simulink model "Main_Model_v0"  (R2025a)
settings: Solver=VariableStepAuto  StartTime=0.0  StopTime=800  RelTol=1e-3  AbsTol=1e-3
values from neighbouring files (symbols this model uses):
  area_air = 0.0353    [air_params.m]
  cp_air = 1005    [air_params.m]
  eta_map = [nan nan nan nan nan nan nan nan nan nan nan nan ... (240 elements, 15x16)]    [motor efficiency map.mat]
  HC_min = 1    [air_params.m]
  HC_nom = 266.43    [air_params.m]
  rho_air = 1.225    [air_params.m]
  speed_bp_rpm = [500 1000 1500 2000 2500 3000 3500 4000 4500 5000 5500 6000 ... (16 elements, 1x16)]    [motor efficiency map.mat]
  torque_bp_Nm = [0 25 50 75 100 125 150 175 200 225 250 275 ... (15 elements, 1x15)]    [motor efficiency map.mat]
  vel_air_nom = 0.18878    [air_params.m]
libraries: fl_lib x26, nesl_utility x14, SimscapeFluids_lib x3
(part 2 of 3)

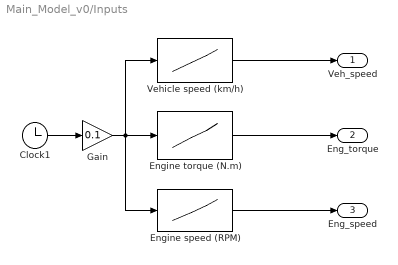
== system Main_Model_v0/Inputs ==
  Clock1 : Clock
  Engine speed (RPM) : Lookup  InputValues=|  Table=|  LookUpMeth=Interpolation-Use End Values
      | [0
      | 1
      | 2
      | 3
      | 4
      | 5
      | 6
      | 7
      | 8
      | 9
      | 10
      | 11
      | 12
      | 13
      | 14
      | 15
      | 16
      | 17
      | 18
      | 19
      | 20
      | 21
      | 22
      | 23
      | 24
      | 25
      | 26
      | 27
      | 28
      | 29
      | 30
      | 31
      | 32
      | 33
      | 34
      | 35
      | 36
      | 37
      | 38
      | 39
      | 40
      | 41
      | 42
      | 43
      | 44
      | 45
      | 46
      | 47
      | 48
      | 49
      | 50
      | 51
      | 52
      | 53
      | 54
      | 55
      | 56
      | 57
      | 58
      | 59
      | 61
      | 62
      | 63
      | 64
      | 65
      | 66
      | 67
      | 68
      | 69
      | 70
      | 71
      | 72
      | 73
      | 74
      | 75
      | 76
      | 77
      | 78
      | 79
      | 80
      | 81
      | 82
      | 83
      | 84
      | 85
      | 86
      | 87
      | 88
      | 89
      | 90
      | 91
      | 92
      | 93
      | 94
      | 95
      | 96
      | 97
      | 98
      | 99
      | 100
      | 101
      | 102
      | 103
      | 104
      | 105
      | 106
      | 107
      | 108
      | 109
      | 110
      | 111
      | 112
      | 113
      | 114
      | 115
      | 116
      | 117
      | 118
      | 119
      | 120
      | 121
      | 122
      | 123
      | 124
      | 125
      | 126
      | 127
      | 129
      | 130
      | 131
      | 132
      | 133
      | 134
      | 135
      | 136
      | 137
      | 138
      | 139
      | 140
      | 141
      | 142
      | 143
      | 144
      | 145
      | 146
      | 147
      | 148
      | 149
      | 150
      | 151
      | 152
      | 153
      | 154
      | 155
      | 156
      | 157
      | 158
      | 159
      | 160
      | 161
      | 162
      | 163
      | 164
      | 165
      | 166
      | 167
      | 168
      | 169
      | 170
      | 171
      | 172
      | 173
      | 174
      | 175
      | 176
      | 177
      | 178
      | 179
      | 180
      | 182
      | 183
      | 184
      | 185
      | 186
      | 187
      | 188
      | 189
      | 190
      | 191
      | 192
      | 193
      | 194
      | 195
      | 196
      | 197
      | 198
      | 199
      | 200
      | 201
      | 202
      | 203
      | 204
      | 205
      | 206
      | 207
      | 208
      | 209
      | 210
      | 211
      | 212
      | 213
      | 214
      | 215
      | 216
      | 217
      | 218
      | 219
      | 220
      | 221
      | 222
      | 223
      | 224
      | 225
      | 226
      | 227
      | 228
      | 229
      | 230
      | 231
      | 232
      | 233
      | 234
      | 235
      | 236
      | 237
      | 238
      | 239
      | 240
      | 241
      | 242
      | 243
      | 244
      | 245
      | 246
      | 247
      | 248
      | 249
      | 250
      | 251
      | 252
      | 253
      | 254
      | 255
      | 256
      | 257
      | 258
      | 259
      | 260
      | 261
      | 262
      | 263
      | 264
      | 265
      | 266
      | 267
      | 268
      | 269
      | 270
      | 271
      | 272
      | 273
      | 274
      | 275
      | 276
      | 277
      | 278
      | 279
      | 280
      | 281
      | 282
      | 283
      | 284
      | 285
      | 286
      | 287
      | 288
      | 289
      | 290
      | 291
      | 292
      | 293
      | 294
      | 295
      | 296
      | 297
      | 298
      | 299
      | 300
      | 301
      | 302
      | 303
      | 304
      | 305
      | 306
      | 307
      | 308
      | 309
      | 310
      | 311
      | 312
      | 313
      | 314
      | 315
      | 316
      | 317
      | 318
      | 319
      | 320
      | 321
      | 322
      | 323
      | 324
      | 325
      | 326
      | 327
      | 328
      | 329
      | 330
      | 331
      | 332
      | 333
      | 335
      | 336
      | 337
      | 338
      | 339
      | 340
      | 341
      | 342
      | 343
      | 344
      | 345
      | 346
      | 347
      | 348
      | 349
      | 350
      | 351
      | 352
      | 353
      | 354
      | 355
      | 356
      | 357
      | 358
      | 359
      | 360
      | 361
      | 362
      | 363
      | 364
      | 365
      | 366
      | 367
      | 368
      | 369
      | 370
      | 371
      | 372
      | 373
      | 374
      | 375
      | 377
      | 378
      | 379
      | 380
      | 381
      | 382
      | 383
      | 384
      | 385
      | 386
      | 387
      | 388
      | 389
      | 390
      | 391
      | 392
      | 393
      | 394
      | 395
      | 396
      | 397
      | 398
      | 399
      | 400
      | 401
      | 402
      | 403
      | 404
      | 405
      | 406
      | 407
      | 408
      | 409
      | 410
      | 411
      | 412
      | 413
      | 414
      | 415
      | 416
      | 417
      | 418
      | 419
      | 420
      | 421
      | 422
      | 423
      | 424
      | 425
      | 426
      | 427
      | 428
      | 429
      | 430
      | 431
      | 432
      | 433
      | 434
      | 435
      | 436
      | 437
      | 438
      | 439
      | 440
      | 441
      | 442
      | 443
      | 444
      | 445
      | 446
      | 447
      | 448
      | 449
      | 450
      | 451
      | 452
      | 453
      | 454
      | 455
      | 456
      | 457
      | 458
      | 459
      | 460
      | 461
      | 462
      | 463
      | 464
      | 465
      | 466
      | 467
      | 468
      | 469
      | 470
      | 471
      | 472
      | 473
      | 474
      | 475
      | 476
      | 477
      | 478
      | 479
      | 480
      | 481
      | 482
      | 483
      | 484
      | 485
      | 486
      | 487
      | 488
      | 489
      | 490
      | 491
      | 492
      | 493
      | 494
      | 495
      | 496
      | 497
      | 498
      | 499
      | 500
      | 501
      | 502
      | 503
      | 504
      | 505
      | 506
      | 507
      | 508
      | 509
      | 510
      | 511
      | 512
      | 513
      | 514
      | 515
      | 516
      | 517
      | 518
      | 519
      | 520
      | 521
      | 522
      | 523
      | 524
      | 525
      | 526
      | 527
      | 528
      | 530
      | 531
      | 532
      | 533
      | 534
      | 535
      | 536
      | 537
      | 538
      | 539
      | 540
      | 541
      | 542
      | 543
      | 544
      | 545
      | 546
      | 547
      | 548
      | 549
      | 550
      | 551
      | 552
      | 553
      | 554
      | 555
      | 556
      | 557
      | 558
      | 559
      | 560
      | 561
      | 562
      | 563
      | 564
      | 565
      | 566
      | 567
      | 568
      | 569
      | 570
      | 572
      | 573
      | 574
      | 575
      | 576
      | 577
      | 578
      | 579
      | 580
      | 581
      | 582
      | 583
      | 584
      | 585
      | 586
      | 587
      | 588
      | 589
      | 590
      | 591
      | 592
      | 593
      | 594
      | 595
      | 596
      | 597
      | 598
      | 599
      | 600
      | 601
      | 602
      | 603
      | 604
      | 605
      | 606
      | 607
      | 608
      | 609
      | 610
      | 611
      | 612
      | 613
      | 614
      | 615
      | 616
      | 617
      | 618
      | 619
      | 620
      | 621
      | 622
      | 623
      | 624
      | 625
      | 626
      | 627
      | 628
      | 629
      | 630
      | 631
      | 632
      | 633
      | 634
      | 635
      | 636
      | 637
      | 638
      | 639
      | 640
      | 641
      | 642
      | 643
      | 644
      | 645
      | 646
      | 647
      | 648
      | 649
      | 650
      | 651
      | 652
      | 653
      | 654
      | 655
      | 656
      | 657
      | 658
      | 659
      | 660
      | 661
      | 662
      | 663
      | 664
      | 665
      | 666
      | 667
      | 668
      | 669
      | 670
      | 671
      | 672
      | 673
      | 674
      | 675
      | 676
      | 677
      | 678
      | 679
      | 680
      | 681
      | 682
      | 683
      | 684
      | 685
      | 686
      | 687
      | 688
      | 689
      | 690
      | 691
      | 692
      | 693
      | 694
      | 695
      | 696
      | 697
      | 698
      | 699
      | 700
      | 701
      | 702
      | 703
      | 704
      | 705
      | 706
      | 707
      | 708
      | 709
      | 710
      | 711
      | 712
      | 713
      | 714
      | 715
      | 716
      | 717
      | 718
      | 719
      | 720
      | 721
      | 722
      | 723
      | 725
      | 726
      | 727
      | 728
      | 729
      | 730
      | 731
      | 732
      | 733
      | 734
      | 735
      | 736
      | 737
      | 738
      | 739
      | 740
      | 741
      | 742
      | 743
      | 744
      | 745
      | 746
      | 747
      | 748
      | 749
      | 750
      | 751
      | 752
      | 753
      | 754
      | 755
      | 756
      | 757
      | 758
      | 759
      | 760
      | 761
      | 762
      | 763
      | 764
      | 765
      | 766
      | 767
      | 768
      | 769
      | 770
      | 771
      | 772
      | 773
      | 774
      | 775
      | 776
      | 777
      | 778
      | 779
      | 780
      | 781
      | 782
      | 783
      | 784
      | 785
      | 786
      | 787
      | 788
      | 789
      | 790
      | 791
      | 792
      | 793
      | 794
      | 795
      | 796
      | 797
      | 798
      | 799
      | 800
      | 801
      | 802
      | 803
      | 804
      | 805
      | 806
      | 807
      | 808
      | 809
      | 810
      | 811
      | 812
      | 813
      | 814
      | 815
      | 816
      | 817
      | 818
      | 819
      | 820
      | 821
      | 823
      | 824
      | 825
      | 826
      | 827
      | 828
      | 829
      | 830
      | 831
      | 833
      | 834
      | 835
      | 836
      | 837
      | 838
      | 839
      | 840
      | 841
      | 842
      | 843
      | 844
      | 845
      | 846
      | 848
      | 849
      | 850
      | 851
      | 852
      | 853
      | 854
      | 855
      | 856
      | 857
      | 858
      | 859
      | 860
      | 861
      | 862
      | 863
      | 864
      | 865
      | 866
      | 867
      | 868
      | 869
      | 870
      | 871
      | 872
      | 873
      | 874
      | 875
      | 876
      | 877
      | 878
      | 879
      | 880
      | 881
      | 882
      | 883
      | 884
      | 885
      | 886
      | 887
      | 888
      | 889
      | 890
      | 891
      | 892
      | 893
      | 894
      | 895
      | 896
      | 897
      | 898
      | 899
      | 901
      | 902
      | 903
      | 904
      | 905
      | 906
      | 907
      | 908
      | 909
      | 910
      | 911
      | 912
      | 913
      | 914
      | 915
      | 916
      | 917
      | 918
      | 919
      | 920
      | 921
      | 922
      | 923
      | 924
      | 925
      | 926
      | 927
      | 928
      | 929
      | 930
      | 931
      | 932
      | 933
      | 934
      | 935
      | 936
      | 937
      | 938
      | 939
      | 940
      | 941
      | 942
      | 943
      | 944
      | 945
      | 946
      | 947
      | 948
      | 949
      | 950
      | 951
      | 952
      | 953
      | 954
      | 955
      | 956
      | 957
      | 958
      | 959
      | 960
      | 961
      | 962
      | 963
      | 964
      | 965
      | 966
      | 967
      | 968
      | 969
      | 970
      | 971
      | 972
      | 973
      | 974
      | 975
      | 976
      | 977
      | 978
      | 979
      | 980
      | 981
      | 982
      | 983
      | 984
      | 985
      | 986
      | 988
      | 989
      | 990
      | 991
      | 992
      | 993
      | 994
      | 995
      | 996
      | 997
      | 998
      | 999
      | 1000
      | 1001
      | 1002
      | 1003
      | 1004
      | 1005
      | 1006
      | 1007
      | 1008
      | 1009
      | 1010
      | 1011
      | 1012
      | 1013
      | 1014
      | 1015
      | 1016
      | 1017
      | 1018
      | 1019
      | 1020
      | 1021
      | 1022
      | 1023
      | 1024
      | 1025
      | 1026
      | 1027
      | 1028
      | 1029
      | 1030
      | 1031
      | 1032
      | 1033
      | 1034
      | 1035
      | 1036
      | 1037
      | 1038
      | 1039
      | 1040
      | 1041
      | 1042
      | 1043
      | 1044
      | 1045
      | 1046
      | 1047
      | 1048
      | 1049
      | 1050
      | 1051
      | 1052
      | 1053
      | 1054
      | 1055
      | 1056
      | 1057
      | 1058
      | 1059
      | 1060
      | 1061
      | 1062
      | 1063
      | 1064
      | 1065
      | 1066
      | 1067
      | 1068
      | 1069
      | 1070
      | 1071
      | 1072
      | 1073
      | 1074
      | 1075
      | 1076
      | 1077
      | 1078
      | 1079
      | 1080
      | 1081
      | 1082
      | 1083
      | 1084
      | 1085
      | 1086
      | 1087
      | 1088
      | 1089
      | 1090
      | 1091
      | 1092
      | 1093
      | 1094
      | 1095
      | 1096
      | 1097
      | 1098
      | 1099
      | 1100
      | 1101
      | 1102
      | 1103
      | 1104
      | 1105
      | 1106
      | 1107
      | 1108
      | 1109
      | 1110
      | 1111
      | 1112
      | 1113
      | 1114
      | 1115
      | 1116
      | 1117
      | 1118
      | 1119
      | 1120
      | 1121
      | 1122
      | 1123
      | 1124
      | 1125
      | 1126
      | 1127
      | 1128
      | 1129
      | 1130
      | 1131
      | 1132
      | 1133
      | 1134
      | 1135
      | 1136
      | 1137
      | 1138
      | 1139
      | 1140
      | 1141
      | 1142
      | 1143
      | 1144
      | 1145
      | 1146
      | 1147
      | 1148
      | 1149
      | 1150
      | 1151
      | 1152
      | 1153
      | 1154
      | 1155
      | 1156
      | 1157
      | 1158
      | 1159
      | 1160
      | 1161
      | 1162
      | 1163
      | 1164
      | 1165
      | 1166
      | 1167
      | 1168
      | 1169
      | 1170
      | 1171
      | 1172
      | 1173
      | 1174
      | 1175
      | 1176
      | 1177
      | 1178
      | 1179
      | 1180
      | 1181
      | 1182
      | 1183
      | 1184
      | 1185
      | 1186
      | 1187
      | 1188
      | 1189
      | 1190
      | 1191
      | 1192
      | 1193
      | 1194
      | 1195
      | 1196
      | 1197
      | 1198
      | 1199
      | 1200
      | 1201
      | 1202
      | 1203
      | 1204
      | 1205]
      | [10
      | 10
      | 10
      | 10
      | 806
      | 1376
      | 1306
      | 1251
      | 1223
      | 1214
      | 1207
      | 1214
      | 1234
      | 1188
      | 1189
      | 1029
      | 1032
      | 978
      | 970
      | 1350
      | 1799
      | 1957
      | 1948
      | 1935
      | 1915
      | 1894
      | 1875
      | 1851
      | 1757
      | 1500
      | 1158
      | 1074
      | 1025
      | 991
      | 973
      | 978
      | 974
      | 970
      | 980
      | 979
      | 972
      | 954
      | 984
      | 975
      | 972
      | 971
      | 976
      | 958
      | 956
      | 963
      | 974
      | 973
      | 963
      | 1017
      | 1026
      | 1043
      | 1036
      | 1300
      | 1752
      | 1910
      | 988
      | 1170
      | 1523
      | 1747
      | 1911
      | 2117
      | 2171
      | 2172
      | 2167
      | 2171
      | 2174
      | 2167
      | 2168
      | 2163
      | 2161
      | 2158
      | 2148
      | 2150
      | 2139
      | 2140
      | 2135
      | 2130
      | 2125
      | 2122
      | 2117
      | 2109
      | 2111
      | 2106
      | 2099
      | 2019
      | 1896
      | 1722
      | 1547
      | 1372
      | 1204
      | 1035
      | 986
      | 963
      | 941
      | 941
      | 935
      | 925
      | 930
      | 919
      | 915
      | 923
      | 922
      | 931
      | 911
      | 926
      | 933
      | 913
      | 917
      | 930
      | 920
      | 915
      | 924
      | 914
      | 916
      | 916
      | 921
      | 932
      | 1028
      | 1015
      | 1282
      | 1742
      | 1900
      | 997
      | 1123
      | 1375
      | 1488
      | 1711
      | 1864
      | 1976
      | 2128
      | 2289
      | 2296
      | 1551
      | 1593
      | 1684
      | 1799
      | 1902
      | 1978
      | 2071
      | 2138
      | 2198
      | 2248
      | 2264
      | 2268
      | 2272
      | 2268
      | 2264
      | 2262
      | 2259
      | 2258
      | 2252
      | 2249
      | 2250
      | 2199
      | 2142
      | 2069
      | 1979
      | 1905
      | 1828
      | 1747
      | 1687
      | 1610
      | 1622
      | 1610
      | 1602
      | 1602
      | 1598
      | 1597
      | 1594
      | 1603
      | 1597
      | 1590
      | 1598
      | 1603
      | 2234
      | 2150
      | 1948
      | 1743
      | 1518
      | 1307
      | 1098
      | 967
      | 933
      | 907
      | 879
      | 873
      | 880
      | 876
      | 875
      | 878
      | 868
      | 871
      | 869
      | 859
      | 854
      | 867
      | 874
      | 873
      | 852
      | 864
      | 867
      | 872
      | 810
      | 795
      | 1005
      | 989
      | 1327
      | 1805
      | 1973
      | 1956
      | 1939
      | 1922
      | 1893
      | 1874
      | 1845
      | 1755
      | 1497
      | 900
      | 877
      | 863
      | 858
      | 869
      | 850
      | 862
      | 856
      | 850
      | 846
      | 858
      | 849
      | 844
      | 858
      | 850
      | 852
      | 863
      | 847
      | 849
      | 855
      | 840
      | 859
      | 855
      | 799
      | 783
      | 1018
      | 1053
      | 1297
      | 1733
      | 1917
      | 1013
      | 952
      | 1184
      | 1515
      | 1756
      | 1911
      | 2105
      | 2170
      | 2172
      | 2174
      | 2172
      | 2175
      | 2166
      | 2167
      | 2165
      | 2161
      | 2156
      | 2148
      | 2148
      | 2138
      | 2142
      | 2137
      | 2130
      | 2124
      | 2121
      | 2113
      | 2107
      | 2112
      | 2105
      | 2099
      | 2030
      | 1895
      | 1717
      | 1551
      | 1367
      | 1200
      | 1024
      | 922
      | 897
      | 867
      | 835
      | 834
      | 815
      | 837
      | 821
      | 820
      | 812
      | 819
      | 823
      | 811
      | 831
      | 819
      | 812
      | 833
      | 825
      | 810
      | 828
      | 824
      | 807
      | 831
      | 821
      | 793
      | 803
      | 1020
      | 1043
      | 1282
      | 1751
      | 1912
      | 994
      | 1000
      | 1132
      | 1358
      | 1524
      | 1704
      | 1850
      | 1994
      | 2125
      | 2282
      | 2295
      | 1590
      | 1688
      | 1780
      | 1885
      | 1983
      | 2065
      | 2136
      | 2204
      | 2255
      | 2260
      | 2266
      | 2266
      | 2269
      | 2269
      | 2266
      | 2258
      | 2262
      | 2259
      | 2250
      | 2246
      | 2212
      | 2123
      | 2057
      | 1983
      | 1906
      | 1840
      | 1765
      | 1684
      | 1616
      | 1622
      | 1603
      | 1599
      | 1606
      | 1599
      | 1592
      | 1603
      | 1597
      | 1595
      | 1592
      | 1604
      | 1595
      | 2223
      | 2144
      | 1955
      | 1726
      | 1522
      | 1313
      | 1105
      | 929
      | 877
      | 831
      | 826
      | 799
      | 797
      | 786
      | 803
      | 788
      | 790
      | 792
      | 788
      | 783
      | 792
      | 793
      | 780
      | 781
      | 793
      | 796
      | 777
      | 801
      | 787
      | 816
      | 970
      | 1021
      | 1317
      | 1807
      | 1976
      | 1951
      | 1934
      | 1919
      | 1889
      | 1871
      | 1851
      | 1758
      | 1497
      | 869
      | 806
      | 784
      | 791
      | 796
      | 786
      | 781
      | 789
      | 793
      | 790
      | 779
      | 794
      | 789
      | 788
      | 785
      | 779
      | 791
      | 784
      | 789
      | 777
      | 782
      | 793
      | 791
      | 790
      | 813
      | 1005
      | 1044
      | 1295
      | 1730
      | 1912
      | 1003
      | 960
      | 1187
      | 1499
      | 1785
      | 1908
      | 2123
      | 2169
      | 2168
      | 2174
      | 2173
      | 2173
      | 2166
      | 2162
      | 2163
      | 2162
      | 2154
      | 2145
      | 2147
      | 2139
      | 2139
      | 2138
      | 2133
      | 2128
      | 2115
      | 2116
      | 2115
      | 2111
      | 2104
      | 2101
      | 2027
      | 1893
      | 1715
      | 1548
      | 1369
      | 1197
      | 1026
      | 884
      | 839
      | 809
      | 800
      | 780
      | 779
      | 782
      | 779
      | 781
      | 780
      | 780
      | 781
      | 781
      | 786
      | 780
      | 773
      | 766
      | 771
      | 775
      | 779
      | 761
      | 778
      | 782
      | 772
      | 794
      | 817
      | 983
      | 1054
      | 1289
      | 1759
      | 1907
      | 992
      | 997
      | 1150
      | 1369
      | 1486
      | 1708
      | 1847
      | 1968
      | 2133
      | 2283
      | 2266
      | 1586
      | 1694
      | 1810
      | 1917
      | 1994
      | 2076
      | 2143
      | 2209
      | 2265
      | 2266
      | 2257
      | 2268
      | 2273
      | 2266
      | 2267
      | 2256
      | 2260
      | 2255
      | 2252
      | 2243
      | 2222
      | 2118
      | 2057
      | 1972
      | 1900
      | 1841
      | 1758
      | 1686
      | 1609
      | 1616
      | 1611
      | 1600
      | 1602
      | 1604
      | 1595
      | 1596
      | 1601
      | 1597
      | 1597
      | 1593
      | 1599
      | 2236
      | 2151
      | 1947
      | 1738
      | 1514
      | 1312
      | 1100
      | 931
      | 848
      | 813
      | 801
      | 791
      | 770
      | 765
      | 774
      | 752
      | 778
      | 757
      | 763
      | 774
      | 750
      | 771
      | 766
      | 754
      | 772
      | 754
      | 762
      | 766
      | 803
      | 812
      | 988
      | 981
      | 1332
      | 1823
      | 1976
      | 1952
      | 1936
      | 1916
      | 1897
      | 1877
      | 1849
      | 1768
      | 1492
      | 839
      | 777
      | 763
      | 753
      | 754
      | 763
      | 764
      | 750
      | 746
      | 743
      | 761
      | 759
      | 758
      | 751
      | 748
      | 767
      | 753
      | 753
      | 768
      | 764
      | 756
      | 770
      | 756
      | 809
      | 811
      | 975
      | 1049
      | 1297
      | 1733
      | 1913
      | 996
      | 958
      | 1178
      | 1511
      | 1786
      | 1917
      | 2120
      | 2170
      | 2173
      | 2174
      | 2170
      | 2172
      | 2164
      | 2165
      | 2167
      | 2164
      | 2157
      | 2146
      | 2152
      | 2135
      | 2140
      | 2136
      | 2131
      | 2131
      | 2121
      | 2113
      | 2112
      | 2110
      | 2105
      | 2097
      | 2035
      | 1882
      | 1713
      | 1551
      | 1374
      | 1207
      | 1034
      | 875
      | 822
      | 790
      | 773
      | 758
      | 742
      | 754
      | 749
      | 750
      | 758
      | 764
      | 746
      | 759
      | 747
      | 756
      | 751
      | 740
      | 741
      | 742
      | 740
      | 733
      | 733
      | 747
      | 757
      | 805
      | 814
      | 975
      | 1050
      | 1239
      | 1725
      | 1905
      | 984
      | 983
      | 1176
      | 1303
      | 1537
      | 1671
      | 1830
      | 1991
      | 2145
      | 2266
      | 2295
      | 1593
      | 1719
      | 1835
      | 1930
      | 2004
      | 2048
      | 2121
      | 2188
      | 2263
      | 2268
      | 2266
      | 2272
      | 2262
      | 2267
      | 2260
      | 2266
      | 2255
      | 2249
      | 2240
      | 2242
      | 2220
      | 2140
      | 2072
      | 1975
      | 1907
      | 1829
      | 1748
      | 1682
      | 1606
      | 1618
      | 1601
      | 1604
      | 1596
      | 1598
      | 1599
      | 1595
      | 1594
      | 1599
      | 1597
      | 1597
      | 1595
      | 1558
      | 2243
      | 2159
      | 1939
      | 1742
      | 1523
      | 1305
      | 1096
      | 925
      | 838
      | 791
      | 781
      | 772
      | 762
      | 755
      | 743
      | 746
      | 750
      | 744
      | 736
      | 747
      | 738
      | 745
      | 751
      | 744
      | 745
      | 756
      | 754
      | 755
      | 760
      | 754
      | 757
      | 753
      | 749
      | 742
      | 751
      | 748
      | 756
      | 829
      | 828
      | 1016
      | 1040
      | 1098
      | 1456
      | 1804
      | 1023
      | 1011
      | 1198
      | 1343
      | 1470
      | 1600
      | 1732
      | 1837
      | 2003
      | 2122
      | 2292
      | 1608
      | 1702
      | 1793
      | 1837
      | 1920
      | 1999
      | 2057
      | 2158
      | 2252
      | 1691
      | 1748
      | 1827
      | 1846
      | 1906
      | 1925
      | 2000
      | 2028
      | 2086
      | 2121
      | 2189
      | 2208
      | 2265
      | 2302
      | 1808
      | 1828
      | 1828
      | 1830
      | 1828
      | 1836
      | 1837
      | 1821
      | 1823
      | 1816
      | 1825
      | 1824
      | 1835
      | 1833
      | 1838
      | 1834
      | 1825
      | 1821
      | 1816
      | 1826
      | 1823
      | 1833
      | 1829
      | 1835
      | 1834
      | 1838
      | 1833
      | 1815
      | 1814
      | 1817
      | 1823
      | 1820
      | 1834
      | 1830
      | 1835
      | 1833
      | 1836
      | 1833
      | 1836
      | 1830
      | 1826
      | 1823
      | 1817
      | 1822
      | 1817
      | 1819
      | 1817
      | 1830
      | 1795
      | 1744
      | 1698
      | 1625
      | 1929
      | 1852
      | 1778
      | 1702
      | 1712
      | 1692
      | 1691
      | 1685
      | 1684
      | 1683
      | 1688
      | 1686
      | 1683
      | 1680
      | 1681
      | 1681
      | 1678
      | 1684
      | 1689
      | 1688
      | 1688
      | 1684
      | 1685
      | 1679
      | 1677
      | 1685
      | 1689
      | 1684
      | 1682
      | 1683
      | 1680
      | 1685
      | 1692
      | 1685
      | 1685
      | 1682
      | 1684
      | 1690
      | 1683
      | 1684
      | 1680
      | 1689
      | 1691
      | 1687
      | 1682
      | 1679
      | 1693
      | 1685
      | 1684
      | 1686
      | 1694
      | 1688
      | 1687
      | 1686
      | 1690
      | 1685
      | 1685
      | 1693
      | 1692
      | 1688
      | 1681
      | 1694
      | 1686
      | 1684
      | 1694
      | 1692
      | 1688
      | 1694
      | 1689
      | 1685
      | 1689
      | 1693
      | 1746
      | 1792
      | 1837
      | 1874
      | 1923
      | 1961
      | 2015
      | 2025
      | 2090
      | 2155
      | 2195
      | 2247
      | 2281
      | 2312
      | 1814
      | 1845
      | 1832
      | 1836
      | 1828
      | 1830
      | 1823
      | 1825
      | 1819
      | 1819
      | 1822
      | 1829
      | 1842
      | 1838
      | 1843
      | 1835
      | 1834
      | 1823
      | 1832
      | 1845
      | 1839
      | 1837
      | 1822
      | 1832
      | 1847
      | 1835
      | 1825
      | 1849
      | 1841
      | 1837
      | 1845
      | 1840
      | 1829
      | 1841
      | 1840
      | 1830
      | 1852
      | 1833
      | 1842
      | 1849
      | 1839
      | 1845
      | 1839
      | 1854
      | 1836
      | 1848
      | 1837
      | 1850
      | 1893
      | 1879
      | 1926
      | 1929
      | 1967
      | 1964
      | 1970
      | 2017
      | 2042
      | 2075
      | 2088
      | 2081
      | 2134
      | 2160
      | 2167
      | 2191
      | 2185
      | 2211
      | 2260
      | 2255
      | 2271
      | 2310
      | 2354
      | 2369
      | 2387
      | 2397
      | 2427
      | 2452
      | 2475
      | 2480
      | 2518
      | 2545
      | 2536
      | 2580
      | 2600
      | 2590
      | 2152
      | 2180
      | 2219
      | 2199
      | 2213
      | 2191
      | 2199
      | 2209
      | 2192
      | 2178
      | 2199
      | 2207
      | 2192
      | 2192
      | 2208
      | 2206
      | 2195
      | 2208
      | 2190
      | 2193
      | 2203
      | 2186
      | 2214
      | 2186
      | 2215
      | 2197
      | 2216
      | 2197
      | 2209
      | 2189
      | 2281
      | 2295
      | 2295
      | 2329
      | 2326
      | 2352
      | 2342
      | 2349
      | 2399
      | 2437
      | 2439
      | 2450
      | 2498
      | 2492
      | 2523
      | 2538
      | 2590
      | 2606
      | 2604
      | 2632
      | 2613
      | 2624
      | 2630
      | 2617
      | 2626
      | 2617
      | 2625
      | 2639
      | 2647
      | 2601
      | 2533
      | 2484
      | 2459
      | 2401
      | 2372
      | 2300
      | 2254
      | 2213
      | 2134
      | 2096
      | 2048
      | 1992
      | 1929
      | 1866
      | 1824
      | 1767
      | 1682
      | 1605
      | 1520
      | 1439
      | 1347
      | 1272
      | 1188
      | 895
      | 829
      | 779
      | 769
      | 774
      | 757
      | 760
      | 760
      | 758
      | 749
      | 747
      | 745
      | 740
      | 741
      | 741
      | 740
      | 752
      | 749
      | 759
      | 763
      | 756
      | 754
      | 762
      | 756
      | 759
      | 752
      | 751
      | 762
      | 758
      | 756
      | 757
      | 758
      | 757
      | 757
      | 756
      | 758
      | 750
      | 758
      | 753
      | 746
      | 754
      | 760
      | 756
      | 752
      | 750
      | 746
      | 751
      | 750
      | 750
      | 760
      | 10]
  Engine torque (N.m) : Lookup  InputValues=|  Table=|  LookUpMeth=Interpolation-Use End Values
      | [0
      | 1
      | 2
      | 3
      | 4
      | 5
      | 6
      | 7
      | 8
      | 9
      | 10
      | 11
      | 12
      | 13
      | 14
      | 15
      | 16
      | 17
      | 18
      | 19
      | 20
      | 21
      | 22
      | 23
      | 24
      | 25
      | 26
      | 27
      | 28
      | 29
      | 30
      | 31
      | 32
      | 33
      | 34
      | 35
      | 36
      | 37
      | 38
      | 39
      | 40
      | 41
      | 42
      | 43
      | 44
      | 45
      | 46
      | 47
      | 48
      | 49
      | 50
      | 51
      | 52
      | 53
      | 54
      | 55
      | 56
      | 57
      | 58
      | 59
      | 61
      | 62
      | 63
      | 64
      | 65
      | 66
      | 67
      | 68
      | 69
      | 70
      | 71
      | 72
      | 73
      | 74
      | 75
      | 76
      | 77
      | 78
      | 79
      | 80
      | 81
      | 82
      | 83
      | 84
      | 85
      | 86
      | 87
      | 88
      | 89
      | 90
      | 91
      | 92
      | 93
      | 94
      | 95
      | 96
      | 97
      | 98
      | 99
      | 100
      | 101
      | 102
      | 103
      | 104
      | 105
      | 106
      | 107
      | 108
      | 109
      | 110
      | 111
      | 112
      | 113
      | 114
      | 115
      | 116
      | 117
      | 118
      | 119
      | 120
      | 121
      | 122
      | 123
      | 124
      | 125
      | 126
      | 127
      | 129
      | 130
      | 131
      | 132
      | 133
      | 134
      | 135
      | 136
      | 137
      | 138
      | 139
      | 140
      | 141
      | 142
      | 143
      | 144
      | 145
      | 146
      | 147
      | 148
      | 149
      | 150
      | 151
      | 152
      | 153
      | 154
      | 155
      | 156
      | 157
      | 158
      | 159
      | 160
      | 161
      | 162
      | 163
      | 164
      | 165
      | 166
      | 167
      | 168
      | 169
      | 170
      | 171
      | 172
      | 173
      | 174
      | 175
      | 176
      | 177
      | 178
      | 179
      | 180
      | 182
      | 183
      | 184
      | 185
      | 186
      | 187
      | 188
      | 189
      | 190
      | 191
      | 192
      | 193
      | 194
      | 195
      | 196
      | 197
      | 198
      | 199
      | 200
      | 201
      | 202
      | 203
      | 204
      | 205
      | 206
      | 207
      | 208
      | 209
      | 210
      | 211
      | 212
      | 213
      | 214
      | 215
      | 216
      | 217
      | 218
      | 219
      | 220
      | 221
      | 222
      | 223
      | 224
      | 225
      | 226
      | 227
      | 228
      | 229
      | 230
      | 231
      | 232
      | 233
      | 234
      | 235
      | 236
      | 237
      | 238
      | 239
      | 240
      | 241
      | 242
      | 243
      | 244
      | 245
      | 246
      | 247
      | 248
      | 249
      | 250
      | 251
      | 252
      | 253
      | 254
      | 255
      | 256
      | 257
      | 258
      | 259
      | 260
      | 261
      | 262
      | 263
      | 264
      | 265
      | 266
      | 267
      | 268
      | 269
      | 270
      | 271
      | 272
      | 273
      | 274
      | 275
      | 276
      | 277
      | 278
      | 279
      | 280
      | 281
      | 282
      | 283
      | 284
      | 285
      | 286
      | 287
      | 288
      | 289
      | 290
      | 291
      | 292
      | 293
      | 294
      | 295
      | 296
      | 297
      | 298
      | 299
      | 300
      | 301
      | 302
      | 303
      | 304
      | 305
      | 306
      | 307
      | 308
      | 309
      | 310
      | 311
      | 312
      | 313
      | 314
      | 315
      | 316
      | 317
      | 318
      | 319
      | 320
      | 321
      | 322
      | 323
      | 324
      | 325
      | 326
      | 327
      | 328
      | 329
      | 330
      | 331
      | 332
      | 333
      | 335
      | 336
      | 337
      | 338
      | 339
      | 340
      | 341
      | 342
      | 343
      | 344
      | 345
      | 346
      | 347
      | 348
      | 349
      | 350
      | 351
      | 352
      | 353
      | 354
      | 355
      | 356
      | 357
      | 358
      | 359
      | 360
      | 361
      | 362
      | 363
      | 364
      | 365
      | 366
      | 367
      | 368
      | 369
      | 370
      | 371
      | 372
      | 373
      | 374
      | 375
      | 377
      | 378
      | 379
      | 380
      | 381
      | 382
      | 383
      | 384
      | 385
      | 386
      | 387
      | 388
      | 389
      | 390
      | 391
      | 392
      | 393
      | 394
      | 395
      | 396
      | 397
      | 398
      | 399
      | 400
      | 401
      | 402
      | 403
      | 404
      | 405
      | 406
      | 407
      | 408
      | 409
      | 410
      | 411
      | 412
      | 413
      | 414
      | 415
      | 416
      | 417
      | 418
      | 419
      | 420
      | 421
      | 422
      | 423
      | 424
      | 425
      | 426
      | 427
      | 428
      | 429
      | 430
      | 431
      | 432
      | 433
      | 434
      | 435
      | 436
      | 437
      | 438
      | 439
      | 440
      | 441
      | 442
      | 443
      | 444
      | 445
      | 446
      | 447
      | 448
      | 449
      | 450
      | 451
      | 452
      | 453
      | 454
      | 455
      | 456
      | 457
      | 458
      | 459
      | 460
      | 461
      | 462
      | 463
      | 464
      | 465
      | 466
      | 467
      | 468
      | 469
      | 470
      | 471
      | 472
      | 473
      | 474
      | 475
      | 476
      | 477
      | 478
      | 479
      | 480
      | 481
      | 482
      | 483
      | 484
      | 485
      | 486
      | 487
      | 488
      | 489
      | 490
      | 491
      | 492
      | 493
      | 494
      | 495
      | 496
      | 497
      | 498
      | 499
      | 500
      | 501
      | 502
      | 503
      | 504
      | 505
      | 506
      | 507
      | 508
      | 509
      | 510
      | 511
      | 512
      | 513
      | 514
      | 515
      | 516
      | 517
      | 518
      | 519
      | 520
      | 521
      | 522
      | 523
      | 524
      | 525
      | 526
      | 527
      | 528
      | 530
      | 531
      | 532
      | 533
      | 534
      | 535
      | 536
      | 537
      | 538
      | 539
      | 540
      | 541
      | 542
      | 543
      | 544
      | 545
      | 546
      | 547
      | 548
      | 549
      | 550
      | 551
      | 552
      | 553
      | 554
      | 555
      | 556
      | 557
      | 558
      | 559
      | 560
      | 561
      | 562
      | 563
      | 564
      | 565
      | 566
      | 567
      | 568
      | 569
      | 570
      | 572
      | 573
      | 574
      | 575
      | 576
      | 577
      | 578
      | 579
      | 580
      | 581
      | 582
      | 583
      | 584
      | 585
      | 586
      | 587
      | 588
      | 589
      | 590
      | 591
      | 592
      | 593
      | 594
      | 595
      | 596
      | 597
      | 598
      | 599
      | 600
      | 601
      | 602
      | 603
      | 604
      | 605
      | 606
      | 607
      | 608
      | 609
      | 610
      | 611
      | 612
      | 613
      | 614
      | 615
      | 616
      | 617
      | 618
      | 619
      | 620
      | 621
      | 622
      | 623
      | 624
      | 625
      | 626
      | 627
      | 628
      | 629
      | 630
      | 631
      | 632
      | 633
      | 634
      | 635
      | 636
      | 637
      | 638
      | 639
      | 640
      | 641
      | 642
      | 643
      | 644
      | 645
      | 646
      | 647
      | 648
      | 649
      | 650
      | 651
      | 652
      | 653
      | 654
      | 655
      | 656
      | 657
      | 658
      | 659
      | 660
      | 661
      | 662
      | 663
      | 664
      | 665
      | 666
      | 667
      | 668
      | 669
      | 670
      | 671
      | 672
      | 673
      | 674
      | 675
      | 676
      | 677
      | 678
      | 679
      | 680
      | 681
      | 682
      | 683
      | 684
      | 685
      | 686
      | 687
      | 688
      | 689
      | 690
      | 691
      | 692
      | 693
      | 694
      | 695
      | 696
      | 697
      | 698
      | 699
      | 700
      | 701
      | 702
      | 703
      | 704
      | 705
      | 706
      | 707
      | 708
      | 709
      | 710
      | 711
      | 712
      | 713
      | 714
      | 715
      | 716
      | 717
      | 718
      | 719
      | 720
      | 721
      | 722
      | 723
      | 725
      | 726
      | 727
      | 728
      | 729
      | 730
      | 731
      | 732
      | 733
      | 734
      | 735
      | 736
      | 737
      | 738
      | 739
      | 740
      | 741
      | 742
      | 743
      | 744
      | 745
      | 746
      | 747
      | 748
      | 749
      | 750
      | 751
      | 752
      | 753
      | 754
      | 755
      | 756
      | 757
      | 758
      | 759
      | 760
      | 761
      | 762
      | 763
      | 764
      | 765
      | 766
      | 767
      | 768
      | 769
      | 770
      | 771
      | 772
      | 773
      | 774
      | 775
      | 776
      | 777
      | 778
      | 779
      | 780
      | 781
      | 782
      | 783
      | 784
      | 785
      | 786
      | 787
      | 788
      | 789
      | 790
      | 791
      | 792
      | 793
      | 794
      | 795
      | 796
      | 797
      | 798
      | 799
      | 800
      | 801
      | 802
      | 803
      | 804
      | 805
      | 806
      | 807
      | 808
      | 809
      | 810
      | 811
      | 812
      | 813
      | 814
      | 815
      | 816
      | 817
      | 818
      | 819
      | 820
      | 821
      | 823
      | 824
      | 825
      | 826
      | 827
      | 828
      | 829
      | 830
      | 831
      | 833
      | 834
      | 835
      | 836
      | 837
      | 838
      | 839
      | 840
      | 841
      | 842
      | 843
      | 844
      | 845
      | 846
      | 848
      | 849
      | 850
      | 851
      | 852
      | 853
      | 854
      | 855
      | 856
      | 857
      | 858
      | 859
      | 860
      | 861
      | 862
      | 863
      | 864
      | 865
      | 866
      | 867
      | 868
      | 869
      | 870
      | 871
      | 872
      | 873
      | 874
      | 875
      | 876
      | 877
      | 878
      | 879
      | 880
      | 881
      | 882
      | 883
      | 884
      | 885
      | 886
      | 887
      | 888
      | 889
      | 890
      | 891
      | 892
      | 893
      | 894
      | 895
      | 896
      | 897
      | 898
      | 899
      | 901
      | 902
      | 903
      | 904
      | 905
      | 906
      | 907
      | 908
      | 909
      | 910
      | 911
      | 912
      | 913
      | 914
      | 915
      | 916
      | 917
      | 918
      | 919
      | 920
      | 921
      | 922
      | 923
      | 924
      | 925
      | 926
      | 927
      | 928
      | 929
      | 930
      | 931
      | 932
      | 933
      | 934
      | 935
      | 936
      | 937
      | 938
      | 939
      | 940
      | 941
      | 942
      | 943
      | 944
      | 945
      | 946
      | 947
      | 948
      | 949
      | 950
      | 951
      | 952
      | 953
      | 954
      | 955
      | 956
      | 957
      | 958
      | 959
      | 960
      | 961
      | 962
      | 963
      | 964
      | 965
      | 966
      | 967
      | 968
      | 969
      | 970
      | 971
      | 972
      | 973
      | 974
      | 975
      | 976
      | 977
      | 978
      | 979
      | 980
      | 981
      | 982
      | 983
      | 984
      | 985
      | 986
      | 988
      | 989
      | 990
      | 991
      | 992
      | 993
      | 994
      | 995
      | 996
      | 997
      | 998
      | 999
      | 1000
      | 1001
      | 1002
      | 1003
      | 1004
      | 1005
      | 1006
      | 1007
      | 1008
      | 1009
      | 1010
      | 1011
      | 1012
      | 1013
      | 1014
      | 1015
      | 1016
      | 1017
      | 1018
      | 1019
      | 1020
      | 1021
      | 1022
      | 1023
      | 1024
      | 1025
      | 1026
      | 1027
      | 1028
      | 1029
      | 1030
      | 1031
      | 1032
      | 1033
      | 1034
      | 1035
      | 1036
      | 1037
      | 1038
      | 1039
      | 1040
      | 1041
      | 1042
      | 1043
      | 1044
      | 1045
      | 1046
      | 1047
      | 1048
      | 1049
      | 1050
      | 1051
      | 1052
      | 1053
      | 1054
      | 1055
      | 1056
      | 1057
      | 1058
      | 1059
      | 1060
      | 1061
      | 1062
      | 1063
      | 1064
      | 1065
      | 1066
      | 1067
      | 1068
      | 1069
      | 1070
      | 1071
      | 1072
      | 1073
      | 1074
      | 1075
      | 1076
      | 1077
      | 1078
      | 1079
      | 1080
      | 1081
      | 1082
      | 1083
      | 1084
      | 1085
      | 1086
      | 1087
      | 1088
      | 1089
      | 1090
      | 1091
      | 1092
      | 1093
      | 1094
      | 1095
      | 1096
      | 1097
      | 1098
      | 1099
      | 1100
      | 1101
      | 1102
      | 1103
      | 1104
      | 1105
      | 1106
      | 1107
      | 1108
      | 1109
      | 1110
      | 1111
      | 1112
      | 1113
      | 1114
      | 1115
      | 1116
      | 1117
      | 1118
      | 1119
      | 1120
      | 1121
      | 1122
      | 1123
      | 1124
      | 1125
      | 1126
      | 1127
      | 1128
      | 1129
      | 1130
      | 1131
      | 1132
      | 1133
      | 1134
      | 1135
      | 1136
      | 1137
      | 1138
      | 1139
      | 1140
      | 1141
      | 1142
      | 1143
      | 1144
      | 1145
      | 1146
      | 1147
      | 1148
      | 1149
      | 1150
      | 1151
      | 1152
      | 1153
      | 1154
      | 1155
      | 1156
      | 1157
      | 1158
      | 1159
      | 1160
      | 1161
      | 1162
      | 1163
      | 1164
      | 1165
      | 1166
      | 1167
      | 1168
      | 1169
      | 1170
      | 1171
      | 1172
      | 1173
      | 1174
      | 1175
      | 1176
      | 1177
      | 1178
      | 1179
      | 1180
      | 1181
      | 1182
      | 1183
      | 1184
      | 1185
      | 1186
      | 1187
      | 1188
      | 1189
      | 1190
      | 1191
      | 1192
      | 1193
      | 1194
      | 1195
      | 1196
      | 1197
      | 1198
      | 1199
      | 1200
      | 1201
      | 1202
      | 1203
      | 1204
      | 1205
      | ]
      | [0
      | 0
      | 0
      | 0
      | -28
      | -43
      | -4
      | -3
      | -2
      | -2
      | -2
      | -2
      | -2
      | -1
      | -1
      | 27
      | 34
      | 37
      | 52
      | 58
      | 32
      | 10
      | 3
      | 3
      | 2
      | 2
      | 3
      | 1
      | -22
      | -16
      | -1
      | -1
      | -1
      | 0
      | -1
      | -1
      | -1
      | -1
      | -1
      | 0
      | -1
      | -1
      | -1
      | 0
      | 0
      | -1
      | -1
      | -1
      | -1
      | 0
      | -1
      | -1
      | -1
      | 5
      | 7
      | 25
      | 28
      | 36
      | 38
      | 15
      | 8
      | 14
      | 34
      | 59
      | 59
      | 58
      | 26
      | 9
      | 8
      | 9
      | 9
      | 8
      | 7
      | 6
      | 7
      | 8
      | 7
      | 7
      | 7
      | 7
      | 6
      | 6
      | 6
      | 6
      | 6
      | 6
      | 6
      | 6
      | 7
      | -26
      | -22
      | -22
      | -21
      | -19
      | -19
      | -2
      | 3
      | -1
      | -2
      | -1
      | -1
      | -1
      | -1
      | -1
      | 0
      | 0
      | -1
      | -1
      | 0
      | -1
      | -2
      | -1
      | -1
      | -1
      | -1
      | -1
      | -1
      | -1
      | -1
      | -1
      | -1
      | -2
      | 20
      | 48
      | 38
      | 47
      | 15
      | 2
      | 33
      | 60
      | 56
      | 58
      | 50
      | 49
      | 48
      | 47
      | 17
      | -9
      | 10
      | 50
      | 69
      | 71
      | 60
      | 55
      | 53
      | 53
      | 53
      | 24
      | 12
      | 13
      | 13
      | 13
      | 13
      | 12
      | 12
      | 13
      | 12
      | 12
      | -27
      | -23
      | -22
      | -22
      | -21
      | -22
      | -21
      | -23
      | -5
      | 16
      | 8
      | 9
      | 9
      | 9
      | 10
      | 10
      | 11
      | 11
      | 10
      | 9
      | 11
      | -24
      | -22
      | -19
      | -19
      | -19
      | -17
      | -16
      | -1
      | -1
      | -2
      | -1
      | -1
      | -1
      | -1
      | -1
      | 0
      | -1
      | -1
      | -1
      | -1
      | -1
      | -1
      | -1
      | -1
      | -1
      | -1
      | -1
      | -2
      | 3
      | 3
      | 23
      | 38
      | 36
      | 45
      | 17
      | -2
      | 4
      | 1
      | 1
      | 1
      | 1
      | -22
      | -16
      | 0
      | -1
      | 0
      | -1
      | 0
      | -1
      | -1
      | -1
      | 0
      | 0
      | -1
      | -1
      | -1
      | -1
      | -1
      | 0
      | -1
      | -1
      | -1
      | 0
      | 0
      | -2
      | 0
      | 3
      | 7
      | 23
      | 38
      | 31
      | 43
      | 18
      | 6
      | 7
      | 28
      | 36
      | 57
      | 55
      | 57
      | 23
      | 8
      | 9
      | 7
      | 8
      | 8
      | 7
      | 6
      | 7
      | 7
      | 7
      | 7
      | 7
      | 6
      | 5
      | 6
      | 6
      | 6
      | 6
      | 6
      | 6
      | 6
      | 6
      | -24
      | -18
      | -18
      | -18
      | -17
      | -16
      | -16
      | 0
      | -1
      | -1
      | -1
      | 0
      | -1
      | 0
      | -1
      | -1
      | -1
      | -1
      | -1
      | -1
      | -1
      | -1
      | -1
      | -1
      | 0
      | -1
      | -1
      | -1
      | -1
      | -1
      | -1
      | 0
      | 2
      | 16
      | 39
      | 33
      | 49
      | 15
      | 6
      | 9
      | 36
      | 62
      | 60
      | 58
      | 52
      | 48
      | 50
      | 48
      | 18
      | 9
      | 48
      | 70
      | 72
      | 59
      | 55
      | 52
      | 52
      | 51
      | 25
      | 11
      | 13
      | 13
      | 12
      | 12
      | 12
      | 11
      | 11
      | 12
      | 11
      | 3
      | -22
      | -19
      | -20
      | -20
      | -20
      | -20
      | -19
      | -3
      | 16
      | 6
      | 10
      | 9
      | 10
      | 9
      | 10
      | 11
      | 11
      | 9
      | 9
      | 9
      | -21
      | -20
      | -17
      | -17
      | -16
      | -16
      | -15
      | -1
      | -2
      | -1
      | -2
      | -1
      | -1
      | 0
      | -1
      | -1
      | -1
      | -1
      | 0
      | -1
      | -1
      | -1
      | -1
      | -1
      | -1
      | -1
      | 0
      | -1
      | 0
      | 1
      | 16
      | 40
      | 33
      | 46
      | 20
      | -1
      | 5
      | 3
      | 3
      | 2
      | 3
      | -14
      | -11
      | -1
      | -1
      | -1
      | 0
      | 0
      | -1
      | -1
      | -1
      | -1
      | 0
      | -1
      | -1
      | 0
      | 0
      | -1
      | -1
      | -1
      | -1
      | -1
      | -1
      | -1
      | -1
      | 0
      | -2
      | 7
      | 24
      | 38
      | 35
      | 48
      | 18
      | 4
      | 6
      | 26
      | 45
      | 61
      | 56
      | 58
      | 26
      | 7
      | 8
      | 8
      | 7
      | 7
      | 7
      | 7
      | 6
      | 6
      | 7
      | 7
      | 7
      | 7
      | 6
      | 6
      | 5
      | 5
      | 7
      | 6
      | 6
      | 6
      | 6
      | -21
      | -18
      | -16
      | -16
      | -15
      | -15
      | -14
      | 0
      | 0
      | 0
      | -1
      | -1
      | -1
      | -2
      | -1
      | -1
      | -1
      | -1
      | -1
      | -1
      | -1
      | 0
      | -2
      | -1
      | -1
      | 0
      | -1
      | -1
      | -1
      | -1
      | -1
      | -14
      | 5
      | 19
      | 39
      | 31
      | 51
      | 21
      | 3
      | 8
      | 31
      | 53
      | 58
      | 57
      | 52
      | 47
      | 48
      | 48
      | 16
      | 10
      | 52
      | 72
      | 72
      | 55
      | 53
      | 54
      | 52
      | 51
      | 24
      | 12
      | 13
      | 13
      | 12
      | 12
      | 11
      | 11
      | 11
      | 11
      | 11
      | 4
      | -20
      | -19
      | -18
      | -19
      | -18
      | -18
      | -17
      | -6
      | 14
      | 9
      | 8
      | 8
      | 8
      | 9
      | 9
      | 9
      | 10
      | 10
      | 9
      | 9
      | -20
      | -18
      | -15
      | -15
      | -16
      | -13
      | -14
      | -5
      | -1
      | -1
      | -1
      | -1
      | -1
      | -1
      | 0
      | -2
      | -1
      | -1
      | -1
      | -1
      | -1
      | 0
      | 0
      | -1
      | 0
      | -1
      | -1
      | 0
      | -1
      | 10
      | 17
      | 36
      | 37
      | 45
      | 21
      | 2
      | 4
      | 3
      | 4
      | 3
      | 2
      | -16
      | -15
      | -3
      | -1
      | -1
      | -1
      | 0
      | -1
      | 0
      | 0
      | -1
      | -1
      | -1
      | 0
      | 0
      | -1
      | 0
      | -1
      | -1
      | -1
      | 0
      | -1
      | 0
      | -1
      | -1
      | 5
      | 3
      | 18
      | 47
      | 30
      | 47
      | 21
      | -5
      | 5
      | 25
      | 41
      | 62
      | 57
      | 58
      | 28
      | 8
      | 9
      | 8
      | 8
      | 7
      | 7
      | 7
      | 7
      | 7
      | 6
      | 6
      | 6
      | 6
      | 7
      | 6
      | 6
      | 6
      | 6
      | 6
      | 6
      | 6
      | 6
      | -17
      | -15
      | -12
      | -14
      | -14
      | -10
      | -9
      | 0
      | 0
      | -1
      | -1
      | -1
      | 0
      | -1
      | -1
      | -1
      | -1
      | 0
      | -1
      | -1
      | -1
      | 0
      | -1
      | -1
      | -1
      | -1
      | -1
      | -1
      | -2
      | -1
      | -1
      | -11
      | 2
      | 14
      | 41
      | 36
      | 50
      | 22
      | -4
      | 5
      | 26
      | 56
      | 62
      | 62
      | 54
      | 47
      | 50
      | 48
      | 17
      | 9
      | 46
      | 75
      | 72
      | 58
      | 55
      | 53
      | 53
      | 53
      | 26
      | 11
      | 14
      | 12
      | 12
      | 11
      | 11
      | 11
      | 10
      | 12
      | 11
      | 3
      | -16
      | -14
      | -17
      | -16
      | -14
      | -17
      | -18
      | -4
      | 14
      | 10
      | 10
      | 10
      | 9
      | 9
      | 10
      | 9
      | 8
      | 9
      | 10
      | 10
      | -19
      | -19
      | -17
      | -16
      | -15
      | -15
      | -14
      | -15
      | 0
      | -1
      | -2
      | -1
      | -1
      | -1
      | -1
      | 0
      | -1
      | -1
      | -1
      | 0
      | -1
      | -1
      | -1
      | -1
      | -1
      | -1
      | -1
      | -1
      | -1
      | -2
      | -1
      | -1
      | -1
      | 0
      | -1
      | 0
      | -1
      | -1
      | 11
      | 7
      | 15
      | 37
      | 28
      | 30
      | 32
      | -9
      | 10
      | 35
      | 41
      | 47
      | 45
      | 46
      | 45
      | 45
      | 46
      | 40
      | 24
      | 50
      | 53
      | 54
      | 55
      | 55
      | 56
      | 55
      | 56
      | 24
      | 56
      | 68
      | 68
      | 68
      | 70
      | 70
      | 69
      | 72
      | 71
      | 73
      | 74
      | 75
      | 53
      | 17
      | 33
      | 34
      | 33
      | 32
      | 33
      | 30
      | 32
      | 30
      | 32
      | 31
      | 31
      | 31
      | 29
      | 32
      | 32
      | 33
      | 30
      | 31
      | 31
      | 32
      | 33
      | 31
      | 32
      | 32
      | 32
      | 31
      | 31
      | 32
      | 33
      | 32
      | 31
      | 32
      | 31
      | 32
      | 32
      | 31
      | 32
      | 32
      | 32
      | 32
      | 32
      | 32
      | 32
      | 32
      | 31
      | 32
      | 32
      | 5
      | -19
      | -17
      | -18
      | -17
      | -17
      | -17
      | -2
      | 22
      | 13
      | 16
      | 16
      | 16
      | 16
      | 16
      | 17
      | 16
      | 16
      | 16
      | 16
      | 16
      | 17
      | 16
      | 18
      | 17
      | 17
      | 17
      | 17
      | 17
      | 16
      | 17
      | 17
      | 16
      | 16
      | 17
      | 16
      | 18
      | 17
      | 17
      | 17
      | 16
      | 17
      | 18
      | 17
      | 17
      | 17
      | 18
      | 18
      | 17
      | 17
      | 17
      | 18
      | 17
      | 16
      | 16
      | 18
      | 18
      | 16
      | 17
      | 17
      | 17
      | 17
      | 17
      | 17
      | 17
      | 17
      | 18
      | 16
      | 17
      | 17
      | 16
      | 17
      | 17
      | 16
      | 17
      | 18
      | 41
      | 66
      | 64
      | 68
      | 65
      | 68
      | 70
      | 69
      | 70
      | 71
      | 71
      | 73
      | 73
      | 46
      | 16
      | 34
      | 34
      | 33
      | 32
      | 34
      | 34
      | 33
      | 31
      | 32
      | 31
      | 32
      | 32
      | 33
      | 32
      | 32
      | 32
      | 31
      | 33
      | 30
      | 33
      | 33
      | 33
      | 33
      | 32
      | 31
      | 32
      | 32
      | 32
      | 33
      | 32
      | 29
      | 32
      | 31
      | 31
      | 33
      | 33
      | 33
      | 32
      | 33
      | 32
      | 33
      | 32
      | 32
      | 32
      | 33
      | 33
      | 31
      | 63
      | 69
      | 69
      | 68
      | 70
      | 71
      | 71
      | 71
      | 72
      | 72
      | 72
      | 73
      | 72
      | 74
      | 76
      | 78
      | 77
      | 78
      | 78
      | 79
      | 78
      | 79
      | 80
      | 80
      | 81
      | 82
      | 81
      | 82
      | 84
      | 83
      | 85
      | 87
      | 85
      | 85
      | 85
      | 62
      | -11
      | 24
      | 57
      | 64
      | 62
      | 62
      | 64
      | 63
      | 62
      | 62
      | 64
      | 63
      | 64
      | 64
      | 64
      | 64
      | 63
      | 64
      | 63
      | 64
      | 63
      | 64
      | 65
      | 63
      | 64
      | 64
      | 62
      | 64
      | 64
      | 60
      | 95
      | 117
      | 112
      | 115
      | 117
      | 117
      | 120
      | 120
      | 120
      | 121
      | 123
      | 121
      | 126
      | 126
      | 124
      | 126
      | 127
      | 130
      | 132
      | 117
      | 92
      | 87
      | 88
      | 85
      | 85
      | 86
      | 84
      | 85
      | 84
      | 60
      | -20
      | -18
      | -18
      | -19
      | -17
      | -17
      | -18
      | -17
      | -17
      | -18
      | -18
      | -17
      | -17
      | -17
      | -17
      | -17
      | -16
      | -15
      | -16
      | -16
      | -15
      | -14
      | -14
      | -1
      | -1
      | -1
      | 0
      | 0
      | -1
      | -1
      | 0
      | 0
      | -1
      | -1
      | -1
      | 0
      | -1
      | 0
      | -1
      | -1
      | 0
      | 0
      | 0
      | -1
      | 0
      | 0
      | -1
      | 0
      | -1
      | -1
      | 0
      | -1
      | 0
      | 0
      | -1
      | -1
      | 0
      | 0
      | -1
      | 0
      | -1
      | 0
      | 0
      | 0
      | -1
      | 0
      | 0
      | 0
      | 0
      | -1
      | 0
      | 0
      | -1
      | 0
      | ]
  Gain : Gain  Gain=0.1
  Vehicle speed (km/h) : Lookup  InputValues=|  Table=|  LookUpMeth=Interpolation-Use End Values
      | [0
      | 1
      | 2
      | 3
      | 4
      | 5
      | 6
      | 7
      | 8
      | 9
      | 10
      | 11
      | 12
      | 13
      | 14
      | 15
      | 16
      | 17
      | 18
      | 19
      | 20
      | 21
      | 22
      | 23
      | 24
      | 25
      | 26
      | 27
      | 28
      | 29
      | 30
      | 31
      | 32
      | 33
      | 34
      | 35
      | 36
      | 37
      | 38
      | 39
      | 40
      | 41
      | 42
      | 43
      | 44
      | 45
      | 46
      | 47
      | 48
      | 49
      | 50
      | 51
      | 52
      | 53
      | 54
      | 55
      | 56
      | 57
      | 58
      | 59
      | 61
      | 62
      | 63
      | 64
      | 65
      | 66
      | 67
      | 68
      | 69
      | 70
      | 71
      | 72
      | 73
      | 74
      | 75
      | 76
      | 77
      | 78
      | 79
      | 80
      | 81
      | 82
      | 83
      | 84
      | 85
      | 86
      | 87
      | 88
      | 89
      | 90
      | 91
      | 92
      | 93
      | 94
      | 95
      | 96
      | 97
      | 98
      | 99
      | 100
      | 101
      | 102
      | 103
      | 104
      | 105
      | 106
      | 107
      | 108
      | 109
      | 110
      | 111
      | 112
      | 113
      | 114
      | 115
      | 116
      | 117
      | 118
      | 119
      | 120
      | 121
      | 122
      | 123
      | 124
      | 125
      | 126
      | 127
      | 129
      | 130
      | 131
      | 132
      | 133
      | 134
      | 135
      | 136
      | 137
      | 138
      | 139
      | 140
      | 141
      | 142
      | 143
      | 144
      | 145
      | 146
      | 147
      | 148
      | 149
      | 150
      | 151
      | 152
      | 153
      | 154
      | 155
      | 156
      | 157
      | 158
      | 159
      | 160
      | 161
      | 162
      | 163
      | 164
      | 165
      | 166
      | 167
      | 168
      | 169
      | 170
      | 171
      | 172
      | 173
      | 174
      | 175
      | 176
      | 177
      | 178
      | 179
      | 180
      | 182
      | 183
      | 184
      | 185
      | 186
      | 187
      | 188
      | 189
      | 190
      | 191
      | 192
      | 193
      | 194
      | 195
      | 196
      | 197
      | 198
      | 199
      | 200
      | 201
      | 202
      | 203
      | 204
      | 205
      | 206
      | 207
      | 208
      | 209
      | 210
      | 211
      | 212
      | 213
      | 214
      | 215
      | 216
      | 217
      | 218
      | 219
      | 220
      | 221
      | 222
      | 223
      | 224
      | 225
      | 226
      | 227
      | 228
      | 229
      | 230
      | 231
      | 232
      | 233
      | 234
      | 235
      | 236
      | 237
      | 238
      | 239
      | 240
      | 241
      | 242
      | 243
      | 244
      | 245
      | 246
      | 247
      | 248
      | 249
      | 250
      | 251
      | 252
      | 253
      | 254
      | 255
      | 256
      | 257
      | 258
      | 259
      | 260
      | 261
      | 262
      | 263
      | 264
      | 265
      | 266
      | 267
      | 268
      | 269
      | 270
      | 271
      | 272
      | 273
      | 274
      | 275
      | 276
      | 277
      | 278
      | 279
      | 280
      | 281
      | 282
      | 283
      | 284
      | 285
      | 286
      | 287
      | 288
      | 289
      | 290
      | 291
      | 292
      | 293
      | 294
      | 295
      | 296
      | 297
      | 298
      | 299
      | 300
      | 301
      | 302
      | 303
      | 304
      | 305
      | 306
      | 307
      | 308
      | 309
      | 310
      | 311
      | 312
      | 313
      | 314
      | 315
      | 316
      | 317
      | 318
      | 319
      | 320
      | 321
      | 322
      | 323
      | 324
      | 325
      | 326
      | 327
      | 328
      | 329
      | 330
      | 331
      | 332
      | 333
      | 335
      | 336
      | 337
      | 338
      | 339
      | 340
      | 341
      | 342
      | 343
      | 344
      | 345
      | 346
      | 347
      | 348
      | 349
      | 350
      | 351
      | 352
      | 353
      | 354
      | 355
      | 356
      | 357
      | 358
      | 359
      | 360
      | 361
      | 362
      | 363
      | 364
      | 365
      | 366
      | 367
      | 368
      | 369
      | 370
      | 371
      | 372
      | 373
      | 374
      | 375
      | 377
      | 378
      | 379
      | 380
      | 381
      | 382
      | 383
      | 384
      | 385
      | 386
      | 387
      | 388
      | 389
      | 390
      | 391
      | 392
      | 393
      | 394
      | 395
      | 396
      | 397
      | 398
      | 399
      | 400
      | 401
      | 402
      | 403
      | 404
      | 405
      | 406
      | 407
      | 408
      | 409
      | 410
      | 411
      | 412
      | 413
      | 414
      | 415
      | 416
      | 417
      | 418
      | 419
      | 420
      | 421
      | 422
      | 423
      | 424
      | 425
      | 426
      | 427
      | 428
      | 429
      | 430
      | 431
      | 432
      | 433
      | 434
      | 435
      | 436
      | 437
      | 438
      | 439
      | 440
      | 441
      | 442
      | 443
      | 444
      | 445
      | 446
      | 447
      | 448
      | 449
      | 450
      | 451
      | 452
      | 453
      | 454
      | 455
      | 456
      | 457
      | 458
      | 459
      | 460
      | 461
      | 462
      | 463
      | 464
      | 465
      | 466
      | 467
      | 468
      | 469
      | 470
      | 471
      | 472
      | 473
      | 474
      | 475
      | 476
      | 477
      | 478
      | 479
      | 480
      | 481
      | 482
      | 483
      | 484
      | 485
      | 486
      | 487
      | 488
      | 489
      | 490
      | 491
      | 492
      | 493
      | 494
      | 495
      | 496
      | 497
      | 498
      | 499
      | 500
      | 501
      | 502
      | 503
      | 504
      | 505
      | 506
      | 507
      | 508
      | 509
      | 510
      | 511
      | 512
      | 513
      | 514
      | 515
      | 516
      | 517
      | 518
      | 519
      | 520
      | 521
      | 522
      | 523
      | 524
      | 525
      | 526
      | 527
      | 528
      | 530
      | 531
      | 532
      | 533
      | 534
      | 535
      | 536
      | 537
      | 538
      | 539
      | 540
      | 541
      | 542
      | 543
      | 544
      | 545
      | 546
      | 547
      | 548
      | 549
      | 550
      | 551
      | 552
      | 553
      | 554
      | 555
      | 556
      | 557
      | 558
      | 559
      | 560
      | 561
      | 562
      | 563
      | 564
      | 565
      | 566
      | 567
      | 568
      | 569
      | 570
      | 572
      | 573
      | 574
      | 575
      | 576
      | 577
      | 578
      | 579
      | 580
      | 581
      | 582
      | 583
      | 584
      | 585
      | 586
      | 587
      | 588
      | 589
      | 590
      | 591
      | 592
      | 593
      | 594
      | 595
      | 596
      | 597
      | 598
      | 599
      | 600
      | 601
      | 602
      | 603
      | 604
      | 605
      | 606
      | 607
      | 608
      | 609
      | 610
      | 611
      | 612
      | 613
      | 614
      | 615
      | 616
      | 617
      | 618
      | 619
      | 620
      | 621
      | 622
      | 623
      | 624
      | 625
      | 626
      | 627
      | 628
      | 629
      | 630
      | 631
      | 632
      | 633
      | 634
      | 635
      | 636
      | 637
      | 638
      | 639
      | 640
      | 641
      | 642
      | 643
      | 644
      | 645
      | 646
      | 647
      | 648
      | 649
      | 650
      | 651
      | 652
      | 653
      | 654
      | 655
      | 656
      | 657
      | 658
      | 659
      | 660
      | 661
      | 662
      | 663
      | 664
      | 665
      | 666
      | 667
      | 668
      | 669
      | 670
      | 671
      | 672
      | 673
      | 674
      | 675
      | 676
      | 677
      | 678
      | 679
      | 680
      | 681
      | 682
      | 683
      | 684
      | 685
      | 686
      | 687
      | 688
      | 689
      | 690
      | 691
      | 692
      | 693
      | 694
      | 695
      | 696
      | 697
      | 698
      | 699
      | 700
      | 701
      | 702
      | 703
      | 704
      | 705
      | 706
      | 707
      | 708
      | 709
      | 710
      | 711
      | 712
      | 713
      | 714
      | 715
      | 716
      | 717
      | 718
      | 719
      | 720
      | 721
      | 722
      | 723
      | 725
      | 726
      | 727
      | 728
      | 729
      | 730
      | 731
      | 732
      | 733
      | 734
      | 735
      | 736
      | 737
      | 738
      | 739
      | 740
      | 741
      | 742
      | 743
      | 744
      | 745
      | 746
      | 747
      | 748
      | 749
      | 750
      | 751
      | 752
      | 753
      | 754
      | 755
      | 756
      | 757
      | 758
      | 759
      | 760
      | 761
      | 762
      | 763
      | 764
      | 765
      | 766
      | 767
      | 768
      | 769
      | 770
      | 771
      | 772
      | 773
      | 774
      | 775
      | 776
      | 777
      | 778
      | 779
      | 780
      | 781
      | 782
      | 783
      | 784
      | 785
      | 786
      | 787
      | 788
      | 789
      | 790
      | 791
      | 792
      | 793
      | 794
      | 795
      | 796
      | 797
      | 798
      | 799
      | 800
      | 801
      | 802
      | 803
      | 804
      | 805
      | 806
      | 807
      | 808
      | 809
      | 810
      | 811
      | 812
      | 813
      | 814
      | 815
      | 816
      | 817
      | 818
      | 819
      | 820
      | 821
      | 823
      | 824
      | 825
      | 826
      | 827
      | 828
      | 829
      | 830
      | 831
      | 833
      | 834
      | 835
      | 836
      | 837
      | 838
      | 839
      | 840
      | 841
      | 842
      | 843
      | 844
      | 845
      | 846
      | 848
      | 849
      | 850
      | 851
      | 852
      | 853
      | 854
      | 855
      | 856
      | 857
      | 858
      | 859
      | 860
      | 861
      | 862
      | 863
      | 864
      | 865
      | 866
      | 867
      | 868
      | 869
      | 870
      | 871
      | 872
      | 873
      | 874
      | 875
      | 876
      | 877
      | 878
      | 879
      | 880
      | 881
      | 882
      | 883
      | 884
      | 885
      | 886
      | 887
      | 888
      | 889
      | 890
      | 891
      | 892
      | 893
      | 894
      | 895
      | 896
      | 897
      | 898
      | 899
      | 901
      | 902
      | 903
      | 904
      | 905
      | 906
      | 907
      | 908
      | 909
      | 910
      | 911
      | 912
      | 913
      | 914
      | 915
      | 916
      | 917
      | 918
      | 919
      | 920
      | 921
      | 922
      | 923
      | 924
      | 925
      | 926
      | 927
      | 928
      | 929
      | 930
      | 931
      | 932
      | 933
      | 934
      | 935
      | 936
      | 937
      | 938
      | 939
      | 940
      | 941
      | 942
      | 943
      | 944
      | 945
      | 946
      | 947
      | 948
      | 949
      | 950
      | 951
      | 952
      | 953
      | 954
      | 955
      | 956
      | 957
      | 958
      | 959
      | 960
      | 961
      | 962
      | 963
      | 964
      | 965
      | 966
      | 967
      | 968
      | 969
      | 970
      | 971
      | 972
      | 973
      | 974
      | 975
      | 976
      | 977
      | 978
      | 979
      | 980
      | 981
      | 982
      | 983
      | 984
      | 985
      | 986
      | 988
      | 989
      | 990
      | 991
      | 992
      | 993
      | 994
      | 995
      | 996
      | 997
      | 998
      | 999
      | 1000
      | 1001
      | 1002
      | 1003
      | 1004
      | 1005
      | 1006
      | 1007
      | 1008
      | 1009
      | 1010
      | 1011
      | 1012
      | 1013
      | 1014
      | 1015
      | 1016
      | 1017
      | 1018
      | 1019
      | 1020
      | 1021
      | 1022
      | 1023
      | 1024
      | 1025
      | 1026
      | 1027
      | 1028
      | 1029
      | 1030
      | 1031
      | 1032
      | 1033
      | 1034
      | 1035
      | 1036
      | 1037
      | 1038
      | 1039
      | 1040
      | 1041
      | 1042
      | 1043
      | 1044
      | 1045
      | 1046
      | 1047
      | 1048
      | 1049
      | 1050
      | 1051
      | 1052
      | 1053
      | 1054
      | 1055
      | 1056
      | 1057
      | 1058
      | 1059
      | 1060
      | 1061
      | 1062
      | 1063
      | 1064
      | 1065
      | 1066
      | 1067
      | 1068
      | 1069
      | 1070
      | 1071
      | 1072
      | 1073
      | 1074
      | 1075
      | 1076
      | 1077
      | 1078
      | 1079
      | 1080
      | 1081
      | 1082
      | 1083
      | 1084
      | 1085
      | 1086
      | 1087
      | 1088
      | 1089
      | 1090
      | 1091
      | 1092
      | 1093
      | 1094
      | 1095
      | 1096
      | 1097
      | 1098
      | 1099
      | 1100
      | 1101
      | 1102
      | 1103
      | 1104
      | 1105
      | 1106
      | 1107
      | 1108
      | 1109
      | 1110
      | 1111
      | 1112
      | 1113
      | 1114
      | 1115
      | 1116
      | 1117
      | 1118
      | 1119
      | 1120
      | 1121
      | 1122
      | 1123
      | 1124
      | 1125
      | 1126
      | 1127
      | 1128
      | 1129
      | 1130
      | 1131
      | 1132
      | 1133
      | 1134
      | 1135
      | 1136
      | 1137
      | 1138
      | 1139
      | 1140
      | 1141
      | 1142
      | 1143
      | 1144
      | 1145
      | 1146
      | 1147
      | 1148
      | 1149
      | 1150
      | 1151
      | 1152
      | 1153
      | 1154
      | 1155
      | 1156
      | 1157
      | 1158
      | 1159
      | 1160
      | 1161
      | 1162
      | 1163
      | 1164
      | 1165
      | 1166
      | 1167
      | 1168
      | 1169
      | 1170
      | 1171
      | 1172
      | 1173
      | 1174
      | 1175
      | 1176
      | 1177
      | 1178
      | 1179
      | 1180
      | 1181
      | 1182
      | 1183
      | 1184
      | 1185
      | 1186
      | 1187
      | 1188
      | 1189
      | 1190
      | 1191
      | 1192
      | 1193
      | 1194
      | 1195
      | 1196
      | 1197
      | 1198
      | 1199
      | 1200
      | 1201
      | 1202
      | 1203
      | 1204
      | 1205
      | ]
      | [0
      | 0
      | 0
      | 0
      | 0
      | 0
      | 0
      | 0
      | 0
      | 0
      | 0
      | 0
      | 0
      | 0
      | 0
      | 0
      | 0
      | 8
      | 8
      | 10
      | 14
      | 15
      | 15
      | 15
      | 15
      | 15
      | 15
      | 14
      | 14
      | 12
      | 0
      | 0
      | 0
      | 0
      | 0
      | 0
      | 0
      | 0
      | 0
      | 0
      | 0
      | 0
      | 0
      | 0
      | 0
      | 0
      | 0
      | 0
      | 0
      | 0
      | 0
      | 0
      | 0
      | 0
      | 8
      | 8
      | 8
      | 10
      | 13
      | 15
      | 15
      | 18
      | 22
      | 27
      | 28
      | 31
      | 32
      | 32
      | 32
      | 32
      | 32
      | 32
      | 32
      | 32
      | 32
      | 32
      | 32
      | 32
      | 32
      | 32
      | 32
      | 32
      | 32
      | 32
      | 31
      | 31
      | 31
      | 31
      | 31
      | 30
      | 28
      | 26
      | 23
      | 21
      | 18
      | 16
      | 15
      | 0
      | 0
      | 0
      | 0
      | 0
      | 0
      | 0
      | 0
      | 0
      | 0
      | 0
      | 0
      | 0
      | 0
      | 0
      | 0
      | 0
      | 0
      | 0
      | 0
      | 0
      | 0
      | 0
      | 0
      | 7
      | 8
      | 8
      | 10
      | 14
      | 15
      | 15
      | 17
      | 20
      | 22
      | 25
      | 27
      | 30
      | 31
      | 33
      | 34
      | 35
      | 35
      | 37
      | 40
      | 42
      | 44
      | 45
      | 47
      | 48
      | 49
      | 50
      | 50
      | 50
      | 50
      | 50
      | 50
      | 49
      | 49
      | 49
      | 49
      | 49
      | 48
      | 47
      | 45
      | 43
      | 42
      | 40
      | 39
      | 37
      | 35
      | 36
      | 35
      | 35
      | 35
      | 35
      | 35
      | 35
      | 35
      | 35
      | 35
      | 35
      | 35
      | 33
      | 32
      | 29
      | 26
      | 23
      | 20
      | 17
      | 0
      | 0
      | 0
      | 0
      | 0
      | 0
      | 0
      | 0
      | 0
      | 0
      | 0
      | 0
      | 0
      | 0
      | 0
      | 0
      | 0
      | 0
      | 0
      | 0
      | 0
      | 0
      | 6
      | 8
      | 8
      | 10
      | 14
      | 15
      | 15
      | 15
      | 15
      | 15
      | 15
      | 14
      | 14
      | 12
      | 0
      | 0
      | 0
      | 0
      | 0
      | 0
      | 0
      | 0
      | 0
      | 0
      | 0
      | 0
      | 0
      | 0
      | 0
      | 0
      | 0
      | 0
      | 0
      | 0
      | 0
      | 0
      | 0
      | 0
      | 6
      | 8
      | 8
      | 10
      | 14
      | 15
      | 15
      | 14
      | 18
      | 22
      | 26
      | 29
      | 31
      | 32
      | 32
      | 32
      | 32
      | 32
      | 32
      | 32
      | 32
      | 32
      | 32
      | 32
      | 32
      | 32
      | 32
      | 32
      | 32
      | 32
      | 32
      | 32
      | 31
      | 31
      | 31
      | 31
      | 30
      | 28
      | 26
      | 23
      | 21
      | 18
      | 15
      | 0
      | 0
      | 0
      | 0
      | 0
      | 0
      | 0
      | 0
      | 0
      | 0
      | 0
      | 0
      | 0
      | 0
      | 0
      | 0
      | 0
      | 0
      | 0
      | 0
      | 0
      | 0
      | 0
      | 0
      | 0
      | 6
      | 7
      | 8
      | 10
      | 13
      | 15
      | 16
      | 14
      | 17
      | 20
      | 23
      | 25
      | 27
      | 30
      | 32
      | 34
      | 34
      | 35
      | 37
      | 39
      | 41
      | 43
      | 45
      | 46
      | 48
      | 49
      | 50
      | 50
      | 50
      | 50
      | 50
      | 49
      | 50
      | 50
      | 49
      | 49
      | 49
      | 49
      | 47
      | 45
      | 44
      | 42
      | 40
      | 38
      | 37
      | 35
      | 36
      | 35
      | 35
      | 35
      | 35
      | 35
      | 35
      | 35
      | 35
      | 35
      | 35
      | 35
      | 33
      | 32
      | 29
      | 26
      | 23
      | 20
      | 17
      | 0
      | 0
      | 0
      | 0
      | 0
      | 0
      | 0
      | 0
      | 0
      | 0
      | 0
      | 0
      | 0
      | 0
      | 0
      | 0
      | 0
      | 0
      | 0
      | 0
      | 0
      | 0
      | 6
      | 8
      | 8
      | 10
      | 14
      | 15
      | 15
      | 15
      | 15
      | 15
      | 15
      | 14
      | 14
      | 12
      | 0
      | 0
      | 0
      | 0
      | 0
      | 0
      | 0
      | 0
      | 0
      | 0
      | 0
      | 0
      | 0
      | 0
      | 0
      | 0
      | 0
      | 0
      | 0
      | 0
      | 0
      | 0
      | 0
      | 0
      | 6
      | 8
      | 8
      | 10
      | 13
      | 15
      | 15
      | 14
      | 18
      | 23
      | 26
      | 29
      | 31
      | 32
      | 32
      | 32
      | 32
      | 32
      | 32
      | 32
      | 32
      | 32
      | 32
      | 32
      | 32
      | 32
      | 32
      | 32
      | 32
      | 32
      | 31
      | 32
      | 31
      | 31
      | 31
      | 31
      | 30
      | 28
      | 26
      | 23
      | 21
      | 18
      | 15
      | 0
      | 0
      | 0
      | 0
      | 0
      | 0
      | 0
      | 0
      | 0
      | 0
      | 0
      | 0
      | 0
      | 0
      | 0
      | 0
      | 0
      | 0
      | 0
      | 0
      | 0
      | 0
      | 0
      | 0
      | 0
      | 6
      | 8
      | 8
      | 10
      | 13
      | 15
      | 15
      | 15
      | 17
      | 19
      | 23
      | 25
      | 27
      | 29
      | 32
      | 34
      | 34
      | 35
      | 38
      | 40
      | 42
      | 43
      | 45
      | 47
      | 48
      | 49
      | 50
      | 50
      | 50
      | 50
      | 50
      | 50
      | 50
      | 49
      | 49
      | 49
      | 49
      | 49
      | 47
      | 45
      | 44
      | 42
      | 40
      | 38
      | 37
      | 35
      | 35
      | 35
      | 35
      | 35
      | 35
      | 35
      | 35
      | 35
      | 35
      | 35
      | 35
      | 35
      | 33
      | 32
      | 29
      | 26
      | 23
      | 20
      | 16
      | 0
      | 0
      | 0
      | 0
      | 0
      | 0
      | 0
      | 0
      | 0
      | 0
      | 0
      | 0
      | 0
      | 0
      | 0
      | 0
      | 0
      | 0
      | 0
      | 0
      | 0
      | 0
      | 6
      | 8
      | 8
      | 10
      | 14
      | 15
      | 15
      | 15
      | 15
      | 15
      | 15
      | 14
      | 14
      | 12
      | 0
      | 0
      | 0
      | 0
      | 0
      | 0
      | 0
      | 0
      | 0
      | 0
      | 0
      | 0
      | 0
      | 0
      | 0
      | 0
      | 0
      | 0
      | 0
      | 0
      | 0
      | 0
      | 0
      | 0
      | 6
      | 8
      | 8
      | 10
      | 14
      | 15
      | 16
      | 14
      | 18
      | 23
      | 26
      | 29
      | 31
      | 32
      | 32
      | 32
      | 32
      | 32
      | 32
      | 32
      | 32
      | 32
      | 32
      | 32
      | 32
      | 32
      | 32
      | 32
      | 32
      | 32
      | 32
      | 31
      | 31
      | 31
      | 31
      | 31
      | 30
      | 28
      | 25
      | 23
      | 21
      | 18
      | 15
      | 0
      | 0
      | 0
      | 0
      | 0
      | 0
      | 0
      | 0
      | 0
      | 0
      | 0
      | 0
      | 0
      | 0
      | 0
      | 0
      | 0
      | 0
      | 0
      | 0
      | 0
      | 0
      | 0
      | 0
      | 0
      | 6
      | 7
      | 8
      | 10
      | 13
      | 15
      | 15
      | 15
      | 17
      | 20
      | 23
      | 24
      | 28
      | 30
      | 31
      | 34
      | 34
      | 35
      | 37
      | 40
      | 41
      | 44
      | 45
      | 47
      | 48
      | 49
      | 49
      | 50
      | 50
      | 50
      | 50
      | 50
      | 50
      | 50
      | 50
      | 49
      | 49
      | 49
      | 47
      | 45
      | 43
      | 42
      | 41
      | 39
      | 37
      | 35
      | 35
      | 35
      | 35
      | 35
      | 35
      | 35
      | 35
      | 35
      | 35
      | 35
      | 35
      | 35
      | 34
      | 33
      | 32
      | 29
      | 26
      | 23
      | 20
      | 17
      | 0
      | 0
      | 0
      | 0
      | 0
      | 0
      | 0
      | 0
      | 0
      | 0
      | 0
      | 0
      | 0
      | 0
      | 0
      | 0
      | 0
      | 0
      | 0
      | 0
      | 0
      | 0
      | 0
      | 0
      | 0
      | 0
      | 0
      | 0
      | 0
      | 0
      | 0
      | 6
      | 8
      | 8
      | 9
      | 11
      | 14
      | 15
      | 15
      | 18
      | 19
      | 22
      | 23
      | 26
      | 28
      | 30
      | 32
      | 34
      | 35
      | 37
      | 39
      | 41
      | 42
      | 44
      | 45
      | 47
      | 49
      | 50
      | 52
      | 54
      | 54
      | 56
      | 57
      | 59
      | 60
      | 61
      | 63
      | 65
      | 66
      | 68
      | 68
      | 69
      | 70
      | 70
      | 69
      | 69
      | 69
      | 70
      | 69
      | 69
      | 69
      | 69
      | 69
      | 69
      | 69
      | 69
      | 69
      | 69
      | 70
      | 70
      | 69
      | 69
      | 70
      | 70
      | 69
      | 69
      | 69
      | 70
      | 70
      | 69
      | 70
      | 69
      | 69
      | 70
      | 69
      | 69
      | 70
      | 69
      | 69
      | 69
      | 69
      | 69
      | 70
      | 69
      | 69
      | 70
      | 70
      | 70
      | 69
      | 68
      | 66
      | 64
      | 63
      | 58
      | 55
      | 53
      | 50
      | 51
      | 50
      | 50
      | 50
      | 50
      | 50
      | 50
      | 50
      | 50
      | 50
      | 50
      | 50
      | 50
      | 50
      | 50
      | 50
      | 50
      | 50
      | 50
      | 50
      | 50
      | 50
      | 50
      | 50
      | 50
      | 50
      | 50
      | 50
      | 50
      | 50
      | 50
      | 50
      | 50
      | 50
      | 50
      | 50
      | 50
      | 50
      | 50
      | 50
      | 50
      | 50
      | 50
      | 50
      | 50
      | 50
      | 50
      | 50
      | 50
      | 50
      | 50
      | 50
      | 50
      | 50
      | 50
      | 50
      | 50
      | 50
      | 50
      | 50
      | 50
      | 50
      | 50
      | 50
      | 50
      | 50
      | 50
      | 50
      | 51
      | 52
      | 53
      | 55
      | 56
      | 58
      | 60
      | 60
      | 62
      | 64
      | 65
      | 66
      | 68
      | 68
      | 69
      | 70
      | 69
      | 69
      | 70
      | 70
      | 69
      | 69
      | 70
      | 70
      | 69
      | 70
      | 70
      | 70
      | 69
      | 69
      | 69
      | 69
      | 70
      | 69
      | 70
      | 70
      | 70
      | 70
      | 70
      | 70
      | 70
      | 69
      | 70
      | 70
      | 70
      | 70
      | 70
      | 69
      | 70
      | 70
      | 69
      | 70
      | 70
      | 70
      | 70
      | 70
      | 70
      | 70
      | 70
      | 70
      | 70
      | 70
      | 71
      | 72
      | 73
      | 73
      | 75
      | 75
      | 76
      | 76
      | 77
      | 77
      | 78
      | 79
      | 81
      | 82
      | 82
      | 83
      | 84
      | 84
      | 85
      | 87
      | 87
      | 87
      | 88
      | 90
      | 90
      | 91
      | 92
      | 93
      | 94
      | 95
      | 96
      | 97
      | 97
      | 98
      | 98
      | 99
      | 98
      | 99
      | 100
      | 100
      | 99
      | 100
      | 100
      | 100
      | 100
      | 100
      | 100
      | 99
      | 99
      | 100
      | 100
      | 100
      | 100
      | 99
      | 100
      | 100
      | 100
      | 100
      | 99
      | 100
      | 99
      | 100
      | 100
      | 101
      | 101
      | 100
      | 103
      | 103
      | 105
      | 104
      | 105
      | 105
      | 108
      | 109
      | 108
      | 111
      | 110
      | 111
      | 112
      | 115
      | 116
      | 116
      | 117
      | 117
      | 118
      | 120
      | 118
      | 118
      | 119
      | 120
      | 119
      | 119
      | 119
      | 119
      | 119
      | 118
      | 114
      | 113
      | 112
      | 110
      | 107
      | 105
      | 102
      | 100
      | 98
      | 96
      | 93
      | 90
      | 87
      | 85
      | 82
      | 80
      | 76
      | 73
      | 69
      | 65
      | 62
      | 58
      | 54
      | 0
      | 0
      | 0
      | 0
      | 0
      | 0
      | 0
      | 0
      | 0
      | 0
      | 0
      | 0
      | 0
      | 0
      | 0
      | 0
      | 0
      | 0
      | 0
      | 0
      | 0
      | 0
      | 0
      | 0
      | 0
      | 0
      | 0
      | 0
      | 0
      | 0
      | 0
      | 0
      | 0
      | 0
      | 0
      | 0
      | 0
      | 0
      | 0
      | 0
      | 0
      | 0
      | 0
      | 0
      | 0
      | 0
      | 0
      | 0
      | 0
      | 0
      | 0
      | ]
  Veh_speed : Outport  VectorParamsAs1DForOutWhenUnconnected=off
  Eng_torque : Outport  Port=2  VectorParamsAs1DForOutWhenUnconnected=off
  Eng_speed : Outport  Port=3  VectorParamsAs1DForOutWhenUnconnected=off
  wires:
  Gain/1 -> Engine speed (RPM)/1, Engine torque (N.m)/1, Vehicle speed (km/h)/1
  Engine torque (N.m)/1 -> Eng_torque/1
  Vehicle speed (km/h)/1 -> Veh_speed/1
  Clock1/1 -> Gain/1
  Engine speed (RPM)/1 -> Eng_speed/1
